simulink model "new"  (R2019a)
settings: Solver=VariableStepAuto  StartTime=0.0  StopTime=stopTime  RelTol=1e-3
undefined symbols (not defined in the file or in its folder): avg_usersArg, lambda1Arg, lambda2Arg, lower_limitArg, random_seedArg, risk_delay_lengthArg, risk_delayArg, upper_limitArg
libraries: rllib x1
settings Model: Creator=Saurav  LastModifiedBy=Saurav

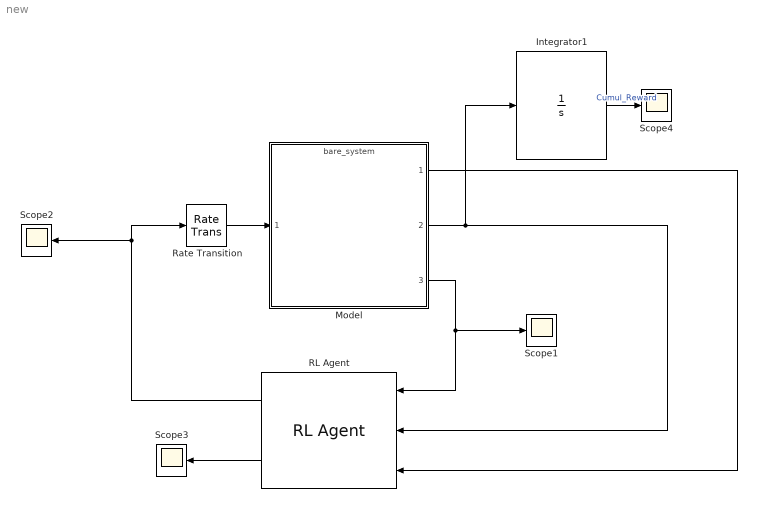
== system new ==
  Integrator1 : Integrator  ZeroCross=off
  Model : ModelReference  ModelNameDialog=bare_system  ParameterArgumentNames=lambda1Arg,lambda2Arg,random_seedArg,avg_usersArg,risk_delayArg,risk_delay_lengthArg,lower_limitArg,upper_limitArg  ParameterArgumentValues=0.74433,9.8611,211287,3,0.65625,3,10,10  UsingDefaultArgumentValue=0,0,0,0,0,0,0,0  SimulationMode=Normal  ModelReferenceVersion=1.148
  RL Agent : rllib/RL Agent  Agent=agent  ProvideReward=on  ProvideIsDone=on  ProvideCumRwd=on  TreatAsDirectFeedthrough=on  CollectLoggedSignals=on  CollectModelStates=on
      settings: SourceProductName=Reinforcement Learning Toolbox
  Rate Transition : RateTransition
  Scope{1..4} (4 alike) : Scope
  wires:
  Model/2 -> Integrator1/1, RL Agent/2
  RL Agent/2 -> Scope3/1
  Model/3 -> RL Agent/1, Scope1/1
  Model/1 -> RL Agent/3
  RL Agent/1 -> Rate Transition/1, Scope2/1
  Integrator1/1 -> Scope4/1  "Cumul_Reward"
  Rate Transition/1 -> Model/1
